simulink model "M1"  (R2024a)
settings: Solver=VariableStepAuto  StartTime=0.0  StopTime=10  RelTol=1e-3
model workspace (MAT data in the model file):
  A = 10
  aaaaa = 0
  f1 = 6.28318530718
  f2 = 15.7079632679
settings Model: Creator=BIDO  LastModifiedBy=BIDO

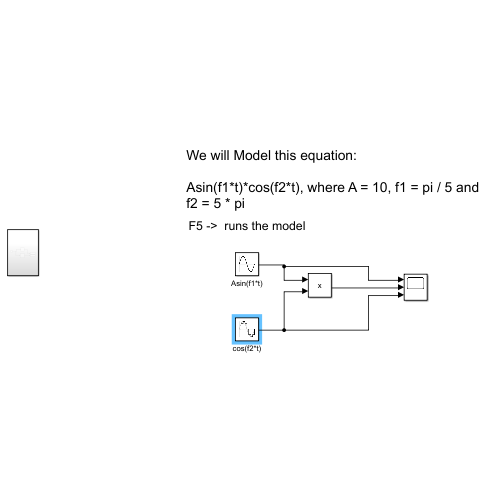
[thumbnail: Simulink's stored preview of the top-level diagram]
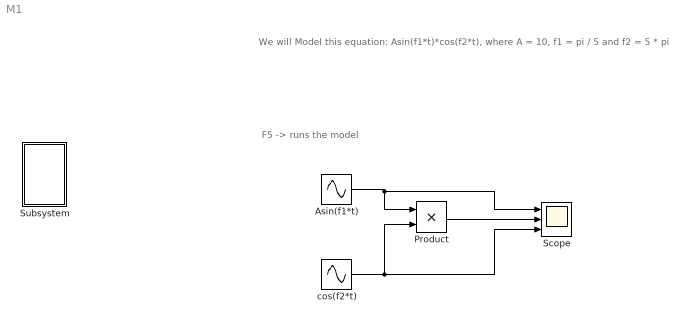
== system M1 ==
  note: We will Model this equation:
      |
      | Asin(f1*t)*cos(f2*t), where A = 10, f1 = pi / 5 and f2 = 5 * pi
  note: F5 -> runs the model
  Asin(f1*t) : Sin  Amplitude=A  Frequency=f1  SampleTime=0
  Product : Product
  Scope : Scope  NumInputPorts=3
  Subsystem : Subsystem
  cos(f2*t) : Sin  Frequency=f2  Phase=pi / 2  SampleTime=0.01
  wires:
  Asin(f1*t)/1 -> Scope/1, Product/1
  cos(f2*t)/1 -> Scope/3, Product/2
  Product/1 -> Scope/2

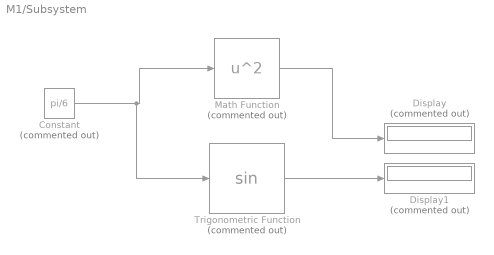
== system M1/Subsystem ==
  Constant : Constant  Commented=on  Value=pi/6
  Display : Display  Commented=on
  Display1 : Display  Commented=on
  Math Function : Math  Commented=on  Operator=square
  Trigonometric Function : Trigonometry  Commented=on
  wires:
  Constant/1 -> Trigonometric Function/1, Math Function/1
  Math Function/1 -> Display/1
  Trigonometric Function/1 -> Display1/1
